simulink model "prodinvsys_sim_mpc"  (R2021b)
settings: Solver=ode15s  StartTime=0.0  StopTime=250  RelTol=1e-3  AbsTol=1e-6
values from neighbouring files (symbols this model uses):
  thetap2 = 1    [run_sim_ol.m]
  Ts = 1    [run_sim_ol.m]    (also in test_prod_inv_sys_dt.m)
undefined symbols (not defined in the file or in its folder): DiscIntNeverNeededParam
libraries: mpclib x1
settings Model: Creator=derivera  LastModifiedBy=billtubbs
settings SolverCC: AutoScaleAbsTol=off  AlgebraicLoopSolver=TrustRegion
settings DataIOCC: SaveFormat=Array  SignalLoggingSaveFormat=ModelDataLogs  ReturnWorkspaceOutputs=off
settings OptimizationCC: BooleanDataType=off  LifeSpan=inf
settings DebuggingCC: SaveWithParameterizedLinksMsg=none  UnderspecifiedInitializationDetection=Classic  MergeDetectMultiDrivingBlocksExec=none  SignalResolutionControl=TryResolveAllWithWarning  MultiTaskDSMMsg=warning  MultiTaskCondExecSysMsg=none  SFUnexpectedBacktrackingDiag=warning  SFNoUnconditionalDefaultTransitionDiag=warning  SFExecutionAtInitializationDiag=none  SFMachineParentedDataDiag=warning  ArithmeticOperatorsInVariantConditions=warning
settings HardwareCC: ProdBitPerPointer=32  ProdBitPerSizeT=32  ProdBitPerPtrDiffT=32  ProdLargestAtomicFloat=None  ProdIntDivRoundTo=Undefined  ProdEndianess=Unspecified  ProdWordSize=32  ProdHWDeviceType=32-bit Generic  TargetUnknown=on
settings ModelReferenceCC: PropagateSignalLabelsOutOfModel=off
settings SFSimCC: SimUseLocalCustomCode=off  CustomCodeUndefinedFunction=UseInterfaceOnly
settings RTWCC: RTWUseLocalCustomCode=off
settings CodeAppCC: StateflowObjectComments=on
settings GRTTargetCC: TargetLangStandard=C89/C90 (ANSI)  CombineOutputUpdateFcns=off  GRTInterface=on
settings ConfigComp: CovMetricSettings=dw  CovSaveCumulativeToWorkspaceVar=on  CovSaveSingleToWorkspaceVar=on  CovExternalEMLEnable=off  CovSFcnEnable=off

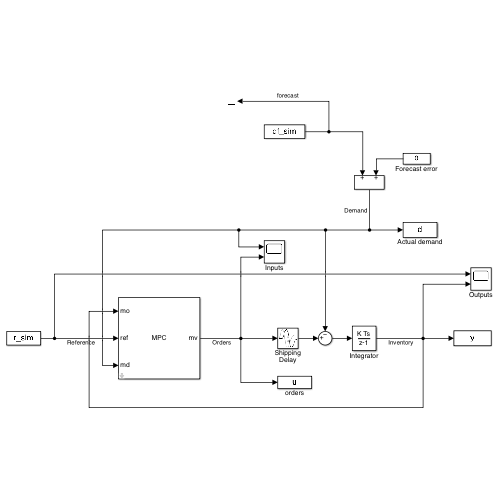
[thumbnail: Simulink's stored preview of the top-level diagram]
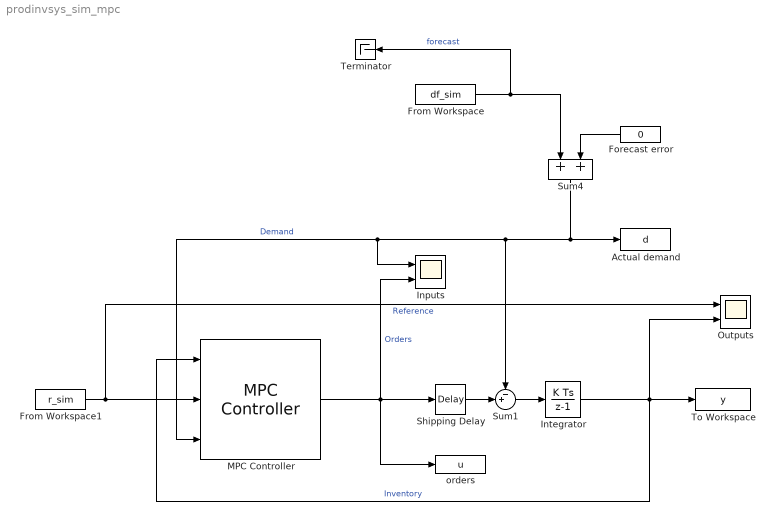
== system prodinvsys_sim_mpc ==
  Actual demand : ToWorkspace  VariableName=d  SampleTime=Ts
  Forecast error : Constant  Value=0
  From Workspace : FromWorkspace  VariableName=df_sim  SampleTime=Ts
  From Workspace1 : FromWorkspace  VariableName=r_sim  SampleTime=Ts
  Inputs : Scope  NumInputPorts=2
  Integrator : DiscreteIntegrator  gainval=1  SampleTime=-1  ICPrevOutput=DiscIntNeverNeededParam  ICPrevScaledInput=DiscIntNeverNeededParam
  MPC Controller : mpclib/MPC Controller  SCDEnableBlockLinearizationSpecification=on  mpcobj=mpcobj  is_multiple=0  enable_value=0  return_u0=off  updateMPCinCallerWorkspace=on  md_inport=on  mv_inport=off  uref_inport=off  return_cost=off  return_mvseq=off  return_qpstatus=off  return_xseq=off  return_state=off  return_ovseq=off  state_inport=off  umin_inport=off  umax_inport=off  ymin_inport=off  ymax_inport=off  cc_inport=off  ywt_inport=off  uwt_inport=off  duwt_inport=off  rhoeps_inport=off  pm_inport=off  MaximumP=10  HorizonChoice=FixedHorizon  n_ts=1  n_p=20  n_mv=1  n_md=1  n_ud=0  n_mo=1  n_uo=0  BlockDataType=double  SampleTimeInherited=off  switch_inport=off
  Outputs : Scope  NumInputPorts=2
  Shipping Delay : TransportDelay  DelayTime=thetap2
  Sum1 : Sum  Inputs=-+|
  Sum4 : Sum  InputSameDT=on  SaturateOnIntegerOverflow=on  OutDataTypeStr=Inherit: Same as first input
  Terminator : Terminator
  To Workspace : ToWorkspace  VariableName=y  SampleTime=Ts
  orders : ToWorkspace  VariableName=u  SampleTime=Ts
  wires:
  From Workspace/1 -> Sum4/1, Terminator/1  "forecast"
  Sum4/1 -> Sum1/1, Inputs/1, MPC Controller/3, Actual demand/1  "Demand"
  Forecast error/1 -> Sum4/2
  Integrator/1 -> MPC Controller/1, To Workspace/1, Outputs/2  "Inventory"
  From Workspace1/1 -> Outputs/1, MPC Controller/2  "Reference"
  Shipping Delay/1 -> Sum1/2
  MPC Controller/1 -> Inputs/2, orders/1, Shipping Delay/1  "Orders"
  Sum1/1 -> Integrator/1
